simulink model "StateFeedback"  (R2022b)
settings: Solver=VariableStepAuto  StartTime=0.0  StopTime=10  RelTol=1e-3
model workspace (MAT data in the model file):
  Sig = Simulink.Signal
  Sig.DataType = 'auto'
  Sig.Dimensions = -1
  Sig.DimensionsMode = 'auto'
  Sig.Complexity = 'auto'
  Sig.SampleTime = -1
  Sig.SamplingMode = 'auto'
values from neighbouring files (symbols this model uses):
  alpha_i = 170 * pi/180    (= 2.96705972839)    [StateFeedbackk.m]
  beta_i = -150 * pi/180    (= -2.61799387799)    [StateFeedbackk.m]
  ka = 10    [StateFeedbackk.m]
  kb = -1.2    [StateFeedbackk.m]
  kp = 5    [StateFeedbackk.m]
  pho_i = 100    [StateFeedbackk.m]
libraries: simulink_extras x6
settings Model: Creator=The MathWorks, Inc.  LastModifiedBy=MuAyman
settings SolverCC: AlgebraicLoopSolver=TrustRegion
settings DebuggingCC: UnconnectedInputMsg=warning  UnconnectedOutputMsg=warning  UnconnectedLineMsg=warning  SymbolicDimsDataTypeCodeGenerationDiagnostic=none  SFMachineParentedDataDiag=warning
settings ModelReferenceCC: EnableRefExpFcnMdlSchedulingChecks=on
settings RTWCC: DLArmComputeVersion=19.05

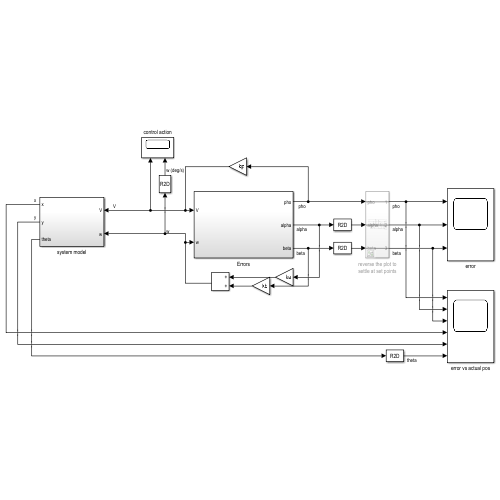
[thumbnail: Simulink's stored preview of the top-level diagram]
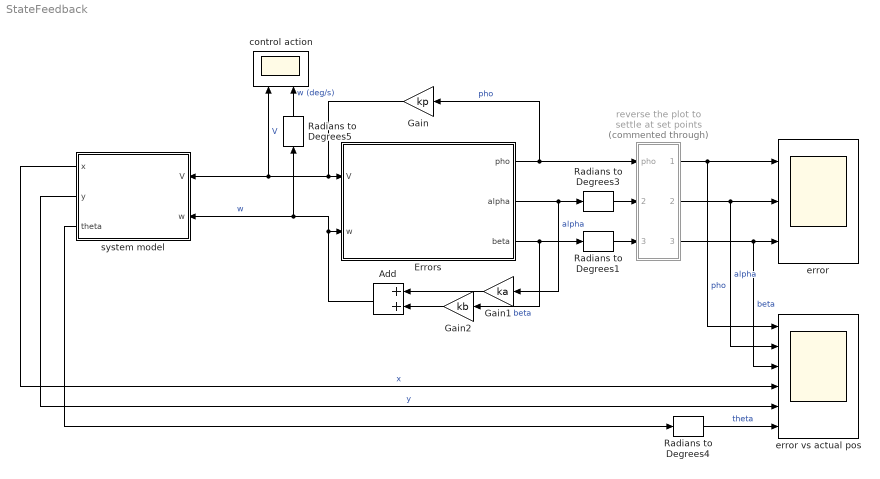
== system StateFeedback ==
  Add : Sum
  Errors : Subsystem
  Gain : Gain  Gain=kp
  Gain1 : Gain  Gain=ka
  Gain2 : Gain  Gain=kb
  Radians to Degrees{1,3..5} (4 alike) : simulink_extras/Transformations/Radians to Degrees
  control action : Scope  NumInputPorts=2
  error : Scope  NumInputPorts=3
  error vs actual pos : Scope  NumInputPorts=6
  reverse the plot to settle at set points : Subsystem  Commented=through
  system model : Subsystem
  wires:
  Errors/1(pho) -> Gain/1, reverse the plot to settle at set points/1(pho)  "pho"
  Errors/2(alpha) -> Gain1/1, Radians to Degrees3/1  "alpha"
  Errors/3(beta) -> Gain2/1, Radians to Degrees1/1  "beta"
  Gain1/1 -> Add/1
  Gain2/1 -> Add/2
  Add/1 -> Radians to Degrees5/1, system model/2(w), Errors/2(w)  "w"
  Gain/1 -> Errors/1(V), system model/1(V), control action/1  "V"
  Radians to Degrees1/1 -> reverse the plot to settle at set points/3(beta)
  Radians to Degrees3/1 -> reverse the plot to settle at set points/2(alpha)
  system model/3(theta) -> Radians to Degrees4/1
  reverse the plot to settle at set points/3(3) -> error vs actual pos/3, error/3  "beta"
  reverse the plot to settle at set points/2(2) -> error vs actual pos/2, error/2  "alpha"
  reverse the plot to settle at set points/1(1) -> error vs actual pos/1, error/1  "pho"
  Radians to Degrees5/1 -> control action/2  "w (deg/s)"
  Radians to Degrees4/1 -> error vs actual pos/6  "theta"
  system model/2(y) -> error vs actual pos/5  "y"
  system model/1(x) -> error vs actual pos/4  "x"

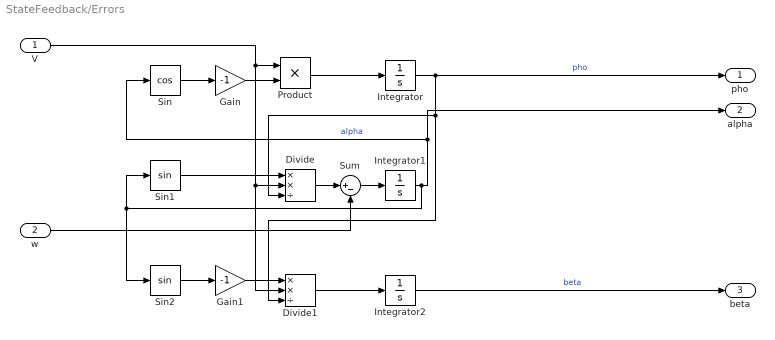
== system StateFeedback/Errors ==
  V : Inport
  w : Inport  Port=2
  Divide : Product  Inputs=**/
  Divide1 : Product  Inputs=**/
  Gain : Gain  Gain=-1
  Gain1 : Gain  Gain=-1
  Integrator : Integrator  InitialCondition=pho_i
  Integrator1 : Integrator  InitialCondition=alpha_i
  Integrator2 : Integrator  InitialCondition=beta_i
  Product : Product
  Sin : Trigonometry  Operator=cos
  Sin1 : Trigonometry
  Sin2 : Trigonometry
  Sum : Sum  Inputs=|+-
  pho : Outport
  alpha : Outport  Port=2
  beta : Outport  Port=3
  wires:
  Integrator1/1 -> alpha/1, Sin/1, Sin2/1, Sin1/1  "alpha"
  V/1 -> Divide1/2, Divide/2, Product/1
  Integrator/1 -> Divide1/3, Divide/3, pho/1  "pho"
  Sin1/1 -> Divide/1
  Sum/1 -> Integrator1/1
  Divide/1 -> Sum/1
  Sin2/1 -> Gain1/1
  Gain/1 -> Product/2
  Sin/1 -> Gain/1
  Product/1 -> Integrator/1
  Gain1/1 -> Divide1/1
  Divide1/1 -> Integrator2/1
  w/1 -> Sum/2
  Integrator2/1 -> beta/1  "beta"

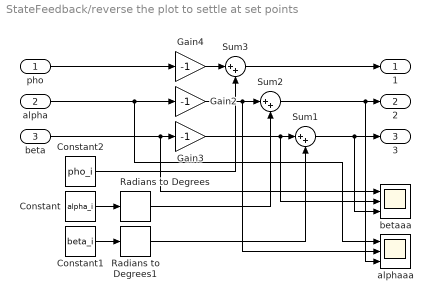
== system StateFeedback/reverse the plot to settle at set points ==
  pho : Inport
  alpha : Inport  Port=2
  beta : Inport  Port=3
  Constant : Constant  Value=alpha_i
  Constant1 : Constant  Value=beta_i
  Constant2 : Constant  Value=pho_i
  Gain2 : Gain  Gain=-1
  Gain3 : Gain  Gain=-1
  Gain4 : Gain  Gain=-1
  Radians to Degrees : simulink_extras/Transformations/Radians to Degrees
  Radians to Degrees1 : simulink_extras/Transformations/Radians to Degrees
  Sum1 : Sum  Inputs=|++
  Sum2 : Sum  Inputs=|++
  Sum3 : Sum  Inputs=|++
  alphaaa : Scope  NumInputPorts=3
  betaaa : Scope  NumInputPorts=3
  1 : Outport
  2 : Outport  Port=2
  3 : Outport  Port=3
  wires:
  alpha/1 -> alphaaa/1, Gain2/1
  Constant2/1 -> Sum3/2
  Constant1/1 -> Radians to Degrees1/1
  Gain4/1 -> Sum3/1
  Constant/1 -> Radians to Degrees/1
  Gain2/1 -> alphaaa/2, Sum2/1
  Gain3/1 -> betaaa/2, Sum1/1
  pho/1 -> Gain4/1
  Sum2/1 -> alphaaa/3, 2/1
  Sum1/1 -> 3/1, betaaa/3
  Sum3/1 -> 1/1
  beta/1 -> betaaa/1, Gain3/1
  Radians to Degrees/1 -> Sum2/2
  Radians to Degrees1/1 -> Sum1/2

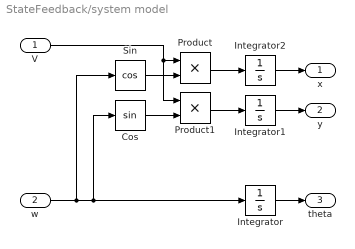
== system StateFeedback/system model ==
  V : Inport
  w : Inport  Port=2
  Cos : Trigonometry
  Integrator : Integrator
  Integrator1 : Integrator
  Integrator2 : Integrator
  Product : Product
  Product1 : Product
  Sin : Trigonometry  Operator=cos
  x : Outport
  y : Outport  Port=2
  theta : Outport  Port=3
  wires:
  Integrator/1 -> theta/1
  w/1 -> Sin/1, Cos/1, Integrator/1
  Sin/1 -> Product/2
  Cos/1 -> Product1/2
  Product1/1 -> Integrator1/1
  Product/1 -> Integrator2/1
  Integrator1/1 -> y/1
  Integrator2/1 -> x/1
  V/1 -> Product1/1, Product/1
